simulink model "DAFC_Quadrotor"  (R2025a)
settings: Solver=VariableStepAuto  StartTime=0.0  StopTime=60  RelTol=1e-3
model workspace (MAT data in the model file):
  gamma_a = Simulink.Parameter
  gamma_a.Value = 100
  gamma_a.Complexity = 'real'
  gamma_a.Dimensions = [1 1]
  gamma_a.DataType = 'auto'
  gamma_p = Simulink.Parameter
  gamma_p.Value = 2.5
  gamma_p.Complexity = 'real'
  gamma_p.Dimensions = [1 1]
  gamma_p.DataType = 'auto'
  pna = Simulink.Parameter
  pna.Value = [3; 3.8]
  pna.Complexity = 'real'
  pna.Dimensions = [2 1]
  pna.DataType = 'auto'
  pnp = Simulink.Parameter
  pnp.Value = [5; 5]
  pnp.Complexity = 'real'
  pnp.Dimensions = [2 1]
  pnp.DataType = 'auto'
values from neighbouring files (symbols this model uses):
  gamma_a = 100    [DAFC_Quadrotor.m]
  gamma_p = 2.5    [DAFC_Quadrotor.m]
  pna = [3;3.8]    [DAFC_Quadrotor.m]
  pnp = [5;5]    [DAFC_Quadrotor.m]
libraries: uavutilslib x1
settings Model: SimulationMode=accelerator  Creator=vinh1  LastModifiedBy=vinh1
settings HardwareCC: ProdBitPerPointer=32.0  ProdBitPerSizeT=32.0  ProdBitPerPtrDiffT=32.0  ProdWordSize=32.0  ProdHWDeviceType=Intel->x86-32 (Windows32)

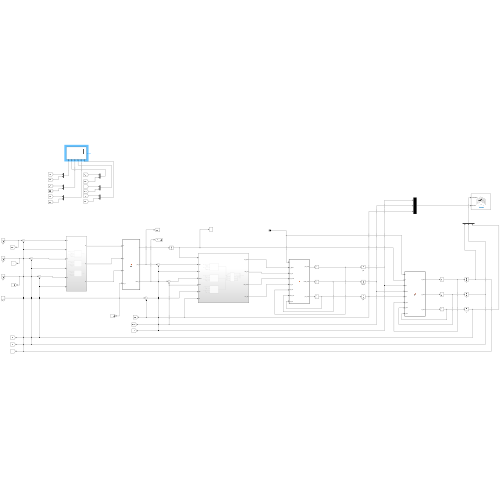
[thumbnail: Simulink's stored preview of the top-level diagram]
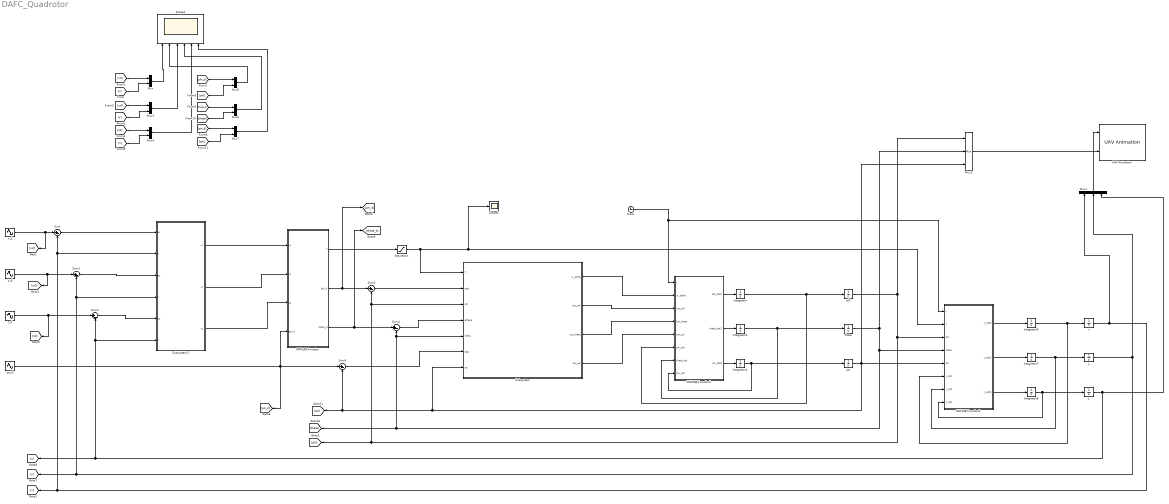
== system DAFC_Quadrotor ==
  Clock : Clock
  Integrator{,2,4,6..8} (6 alike) : Integrator
  MATLAB Function : MATLAB Function  TreatAsAtomicUnit=on
  MATLAB Function1 : MATLAB Function  TreatAsAtomicUnit=on
  MATLAB Function3 : MATLAB Function  TreatAsAtomicUnit=on
  Mux{,3..7} (6 alike) : Mux  Inputs=2
  Mux1 : Mux  Inputs=3
  Mux2 : Mux  Inputs=3
  Saturation : Saturate  UpperLimit=50
  Scope1 : Scope  NumInputPorts=6
      settings: ActiveDisplayString=6  ActiveDisplayYMinimum=-7.5121189989002386E-7  ActiveDisplayYMaximum=4.1251243389959757E-6
  Scope6 : Scope
      settings: ActiveDisplayYMinimum=9.3903851355115471  ActiveDisplayYMaximum=11.595791299111241  DataLoggingVariableName=ScopeData6
  Subsystem : Subsystem
  Subsystem2 : Subsystem
  Sum{,1..5} (6 alike) : Sum  Inputs=|+-
  UAV Animation : uavutilslib/UAV Animation  NumUAV=1  DynamicUAVConfig=off  UAVType=Multirotor  UAVSize=1  UAVColor=[1 0 0]  UAVTrajectoryAlpha=1  InertialZDirection=Up  RotationFormat=Euler ZYX  DrawMarkers=off  SampleTime=-1
  phi : Integrator
  psi : Integrator
  psi_d : Sin  Amplitude=0  Frequency=pi/10  Phase=pi/2  SampleTime=0
  theta : Integrator
  x : Integrator
  x_d : Sin  Amplitude=0.5  Frequency=pi/20  Phase=pi/2  SampleTime=0
  y : Integrator
  y_d : Sin  Amplitude=0.5  Frequency=pi/20  SampleTime=0
  z : Integrator  InitialCondition=2
  z_d : Sin  Amplitude=0.5  Bias=2  Frequency=pi/20  Phase=3*pi/2  SampleTime=0
  wires:
  [psi] -> Mux7/2
  Sum/1 -> Subsystem2/1(ex)
  [phi] -> Mux5/2
  Mux7/1 -> Scope1/6
  Sum2/1 -> Subsystem2/5(ez)
  x_d/1 -> [xd], Sum/1
  Mux6/1 -> Scope1/4
  [zd] -> Mux4/1
  [theta] -> Mux6/2
  Subsystem2/3(uz) -> MATLAB Function/3(uz)
  [yd] -> Mux3/1
  Subsystem2/1(ux) -> MATLAB Function/1(ux)
  [psi_d] -> Mux7/1
  [theta_d] -> Mux6/1
  psi_d/1 -> Sum5/1, [psi_d], MATLAB Function/4(psi_d)
  Subsystem2/2(uy) -> MATLAB Function/2(uy)
  Mux4/1 -> Scope1/5
  [z] -> Mux4/2
  Mux5/1 -> Scope1/2
  [phi_d] -> Mux5/1
  Sum1/1 -> Subsystem2/3(ey)
  Mux3/1 -> Scope1/3
  Mux1/1 -> UAV Animation/1
  [y] -> Mux3/2
  y_d/1 -> Sum1/1, [yd]
  Mux2/1 -> UAV Animation/2
  Mux/1 -> Scope1/1
  z_d/1 -> [zd], Sum2/1
  MATLAB Function1/3(psi_dot2) -> Integrator4/1
  MATLAB Function1/2(theta_dot2) -> Integrator2/1
  MATLAB Function1/1(phi_dot2) -> Integrator/1
  Integrator/1 -> phi/1, MATLAB Function1/6(phi_dot)
  Integrator2/1 -> MATLAB Function1/7(theta_dot), theta/1
  Integrator4/1 -> psi/1, MATLAB Function1/8(psi_dot)
  MATLAB Function/2(phi_d) -> Sum3/1, [phi_d]
  MATLAB Function/3(theta_d) -> [theta_d], Sum4/1
  Subsystem/1(w_alpha) -> MATLAB Function1/2(w_alpha)
  Subsystem/2(tau_phi) -> MATLAB Function1/3(tau_phi)
  Subsystem/3(tau_theta) -> MATLAB Function1/4(tau_theta)
  Subsystem/4(tau_psi) -> MATLAB Function1/5(tau_psi)
  Sum3/1 -> Subsystem/2(ephi)
  Sum4/1 -> Subsystem/4(etheta)
  phi/1 -> Mux2/1, Sum3/2, Subsystem/3(phi), [phi], MATLAB Function3/3(phi)
  theta/1 -> Mux2/2, Sum4/2, Subsystem/5(theta), [theta], MATLAB Function3/4(theta)
  psi/1 -> Mux2/3, MATLAB Function3/5(psi), Sum5/2, [psi], Subsystem/7(psi)
  Sum5/1 -> Subsystem/6(epsi)
  MATLAB Function3/3(z_dot2) -> Integrator8/1
  MATLAB Function3/2(y_dot2) -> Integrator7/1
  MATLAB Function3/1(x_dot2) -> Integrator6/1
  Integrator8/1 -> z/1, MATLAB Function3/8(z_dot)
  Integrator7/1 -> MATLAB Function3/7(y_dot), y/1
  Integrator6/1 -> MATLAB Function3/6(x_dot), x/1
  z/1 -> Mux1/3, [z], Sum2/2, Subsystem2/6(z)
  y/1 -> Sum1/2, Subsystem2/4(y), [y], Mux1/2
  x/1 -> Mux1/1, [x], Sum/2, Subsystem2/2(x)
  Clock/1 -> MATLAB Function3/1(t), MATLAB Function1/1(t)
  Saturation/1 -> Scope6/1, MATLAB Function3/2(T), Subsystem/1(T)
  MATLAB Function/1(T) -> Saturation/1
  [xd] -> Mux/1
  [x] -> Mux/2

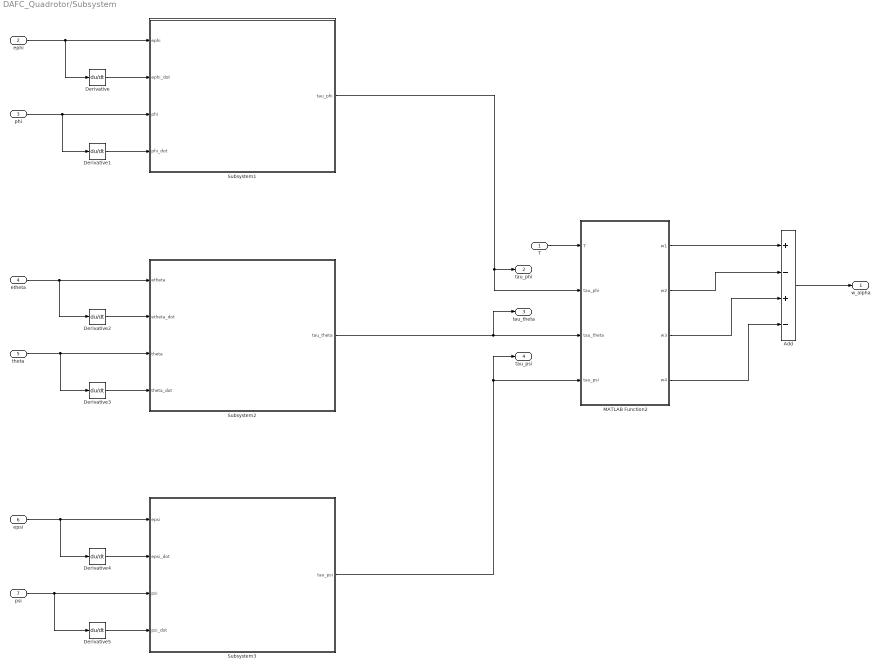
== system DAFC_Quadrotor/Subsystem ==
  T : Inport
  ephi : Inport  Port=2
  phi : Inport  Port=3
  etheta : Inport  Port=4
  theta : Inport  Port=5
  epsi : Inport  Port=6
  psi : Inport  Port=7
  Add : Sum  Inputs=+-+-
  Derivative{,1..5} (6 alike) : Derivative
  MATLAB Function2 : MATLAB Function  TreatAsAtomicUnit=on
  Subsystem1 : Subsystem
  Subsystem2 : Subsystem
  Subsystem3 : Subsystem
  w_alpha : Outport
  tau_phi : Outport  Port=2
  tau_theta : Outport  Port=3
  tau_psi : Outport  Port=4
  wires:
  Derivative4/1 -> Subsystem3/2(epsi_dot)
  Derivative1/1 -> Subsystem1/4(phi_dot)
  Derivative3/1 -> Subsystem2/4(theta_dot)
  Derivative/1 -> Subsystem1/2(ephi_dot)
  Derivative2/1 -> Subsystem2/2(etheta_dot)
  Derivative5/1 -> Subsystem3/4(psi_dot)
  ephi/1 -> Derivative/1, Subsystem1/1(ephi)
  phi/1 -> Subsystem1/3(phi), Derivative1/1
  etheta/1 -> Derivative2/1, Subsystem2/1(etheta)
  theta/1 -> Subsystem2/3(theta), Derivative3/1
  epsi/1 -> Subsystem3/1(epsi), Derivative4/1
  psi/1 -> Derivative5/1, Subsystem3/3(psi)
  MATLAB Function2/3(w3) -> Add/3
  MATLAB Function2/4(w4) -> Add/4
  MATLAB Function2/2(w2) -> Add/2
  MATLAB Function2/1(w1) -> Add/1
  Subsystem1/1(tau_phi) -> tau_phi/1, MATLAB Function2/2(tau_phi)
  Subsystem2/1(tau_theta) -> tau_theta/1, MATLAB Function2/3(tau_theta)
  Subsystem3/1(tau_psi) -> tau_psi/1, MATLAB Function2/4(tau_psi)
  T/1 -> MATLAB Function2/1(T)
  Add/1 -> w_alpha/1

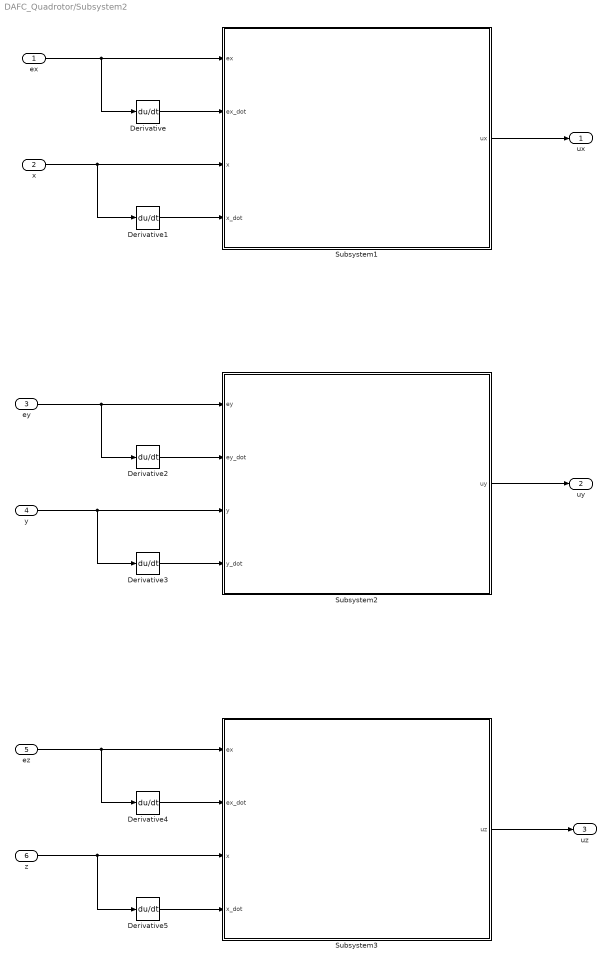
== system DAFC_Quadrotor/Subsystem2 ==
  ex : Inport
  x : Inport  Port=2
  ey : Inport  Port=3
  y : Inport  Port=4
  ez : Inport  Port=5
  z : Inport  Port=6
  Derivative{,1..5} (6 alike) : Derivative
  Subsystem1 : Subsystem
  Subsystem2 : Subsystem
  Subsystem3 : Subsystem
  ux : Outport
  uy : Outport  Port=2
  uz : Outport  Port=3
  wires:
  ex/1 -> Derivative/1, Subsystem1/1(ex)
  Derivative/1 -> Subsystem1/2(ex_dot)
  x/1 -> Subsystem1/3(x), Derivative1/1
  Derivative1/1 -> Subsystem1/4(x_dot)
  ey/1 -> Derivative2/1, Subsystem2/1(ey)
  Derivative2/1 -> Subsystem2/2(ey_dot)
  y/1 -> Subsystem2/3(y), Derivative3/1
  Derivative3/1 -> Subsystem2/4(y_dot)
  ez/1 -> Derivative4/1, Subsystem3/1(ex)
  Derivative4/1 -> Subsystem3/2(ex_dot)
  z/1 -> Derivative5/1, Subsystem3/3(x)
  Derivative5/1 -> Subsystem3/4(x_dot)
  Subsystem1/1(ux) -> ux/1
  Subsystem2/1(uy) -> uy/1
  Subsystem3/1(uz) -> uz/1

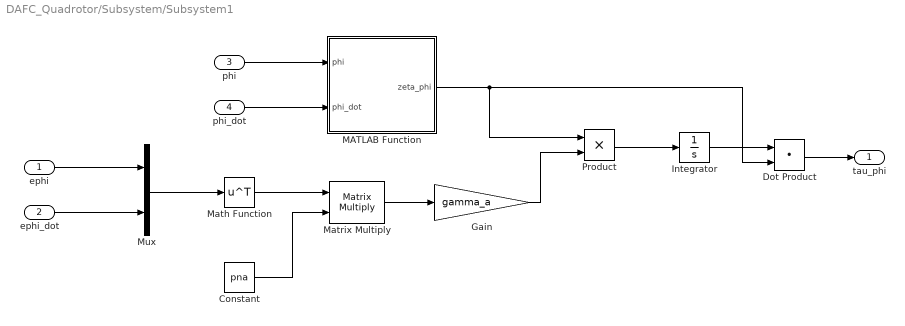
== system DAFC_Quadrotor/Subsystem/Subsystem1 ==
  ephi : Inport
  ephi_dot : Inport  Port=2
  phi : Inport  Port=3
  phi_dot : Inport  Port=4
  Constant : Constant  Value=pna
  Dot Product : DotProduct  OutDataTypeStr=Inherit: Inherit via internal rule
  Gain : Gain  Gain=gamma_a
  Integrator : Integrator
  MATLAB Function : MATLAB Function  TreatAsAtomicUnit=on
  Math Function : Math  Operator=transpose
  Matrix Multiply : Product  Multiplication=Matrix(*)
  Mux : Mux  Inputs=2
  Product : Product
  tau_phi : Outport
  wires:
  Dot Product/1 -> tau_phi/1
  phi_dot/1 -> MATLAB Function/2(phi_dot)
  MATLAB Function/1(zeta_phi) -> Dot Product/2, Product/1
  phi/1 -> MATLAB Function/1(phi)
  Mux/1 -> Math Function/1
  Matrix Multiply/1 -> Gain/1
  Gain/1 -> Product/2
  Constant/1 -> Matrix Multiply/2
  Product/1 -> Integrator/1
  Integrator/1 -> Dot Product/1
  Math Function/1 -> Matrix Multiply/1
  ephi_dot/1 -> Mux/2
  ephi/1 -> Mux/1

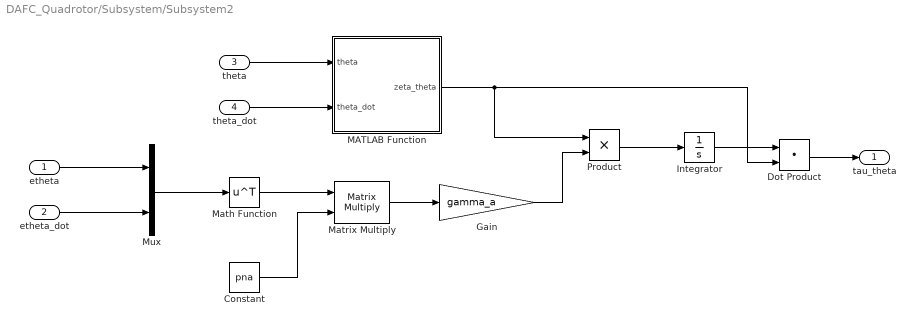
== system DAFC_Quadrotor/Subsystem/Subsystem2 ==
  etheta : Inport
  etheta_dot : Inport  Port=2
  theta : Inport  Port=3
  theta_dot : Inport  Port=4
  Constant : Constant  Value=pna
  Dot Product : DotProduct  OutDataTypeStr=Inherit: Inherit via internal rule
  Gain : Gain  Gain=gamma_a
  Integrator : Integrator
  MATLAB Function : MATLAB Function  TreatAsAtomicUnit=on
  Math Function : Math  Operator=transpose
  Matrix Multiply : Product  Multiplication=Matrix(*)
  Mux : Mux  Inputs=2
  Product : Product
  tau_theta : Outport
  wires:
  etheta/1 -> Mux/1
  etheta_dot/1 -> Mux/2
  Mux/1 -> Math Function/1
  Math Function/1 -> Matrix Multiply/1
  Constant/1 -> Matrix Multiply/2
  Matrix Multiply/1 -> Gain/1
  Gain/1 -> Product/2
  theta/1 -> MATLAB Function/1(theta)
  theta_dot/1 -> MATLAB Function/2(theta_dot)
  Product/1 -> Integrator/1
  MATLAB Function/1(zeta_theta) -> Dot Product/2, Product/1
  Integrator/1 -> Dot Product/1
  Dot Product/1 -> tau_theta/1

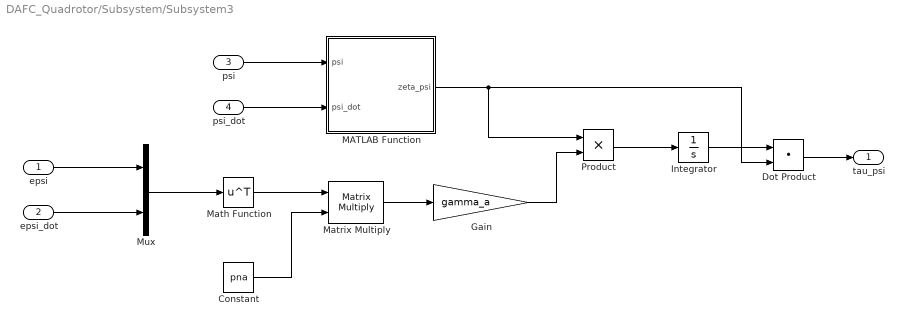
== system DAFC_Quadrotor/Subsystem/Subsystem3 ==
  epsi : Inport
  epsi_dot : Inport  Port=2
  psi : Inport  Port=3
  psi_dot : Inport  Port=4
  Constant : Constant  Value=pna
  Dot Product : DotProduct  OutDataTypeStr=Inherit: Inherit via internal rule
  Gain : Gain  Gain=gamma_a
  Integrator : Integrator
  MATLAB Function : MATLAB Function  TreatAsAtomicUnit=on
  Math Function : Math  Operator=transpose
  Matrix Multiply : Product  Multiplication=Matrix(*)
  Mux : Mux  Inputs=2
  Product : Product
  tau_psi : Outport
  wires:
  Dot Product/1 -> tau_psi/1
  psi_dot/1 -> MATLAB Function/2(psi_dot)
  MATLAB Function/1(zeta_psi) -> Dot Product/2, Product/1
  psi/1 -> MATLAB Function/1(psi)
  Mux/1 -> Math Function/1
  Matrix Multiply/1 -> Gain/1
  Gain/1 -> Product/2
  Constant/1 -> Matrix Multiply/2
  Product/1 -> Integrator/1
  Integrator/1 -> Dot Product/1
  Math Function/1 -> Matrix Multiply/1
  epsi_dot/1 -> Mux/2
  epsi/1 -> Mux/1

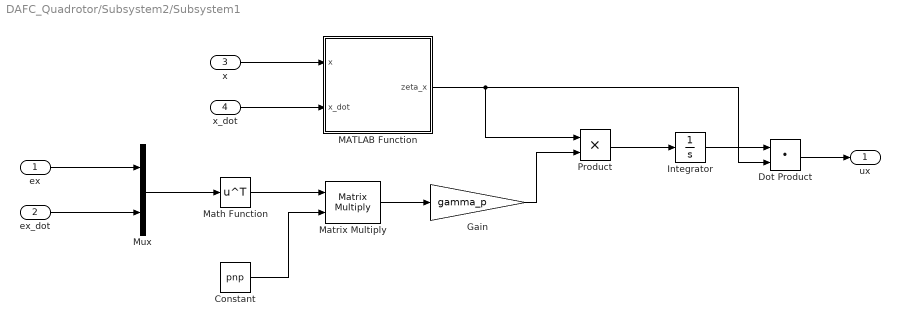
== system DAFC_Quadrotor/Subsystem2/Subsystem1 ==
  ex : Inport
  ex_dot : Inport  Port=2
  x : Inport  Port=3
  x_dot : Inport  Port=4
  Constant : Constant  Value=pnp
  Dot Product : DotProduct  OutDataTypeStr=Inherit: Inherit via internal rule
  Gain : Gain  Gain=gamma_p
  Integrator : Integrator
  MATLAB Function : MATLAB Function  TreatAsAtomicUnit=on
  Math Function : Math  Operator=transpose
  Matrix Multiply : Product  Multiplication=Matrix(*)
  Mux : Mux  Inputs=2
  Product : Product
  ux : Outport
  wires:
  Dot Product/1 -> ux/1
  x_dot/1 -> MATLAB Function/2(x_dot)
  MATLAB Function/1(zeta_x) -> Dot Product/2, Product/1
  x/1 -> MATLAB Function/1(x)
  Mux/1 -> Math Function/1
  Matrix Multiply/1 -> Gain/1
  Gain/1 -> Product/2
  Constant/1 -> Matrix Multiply/2
  Product/1 -> Integrator/1
  Integrator/1 -> Dot Product/1
  Math Function/1 -> Matrix Multiply/1
  ex_dot/1 -> Mux/2
  ex/1 -> Mux/1

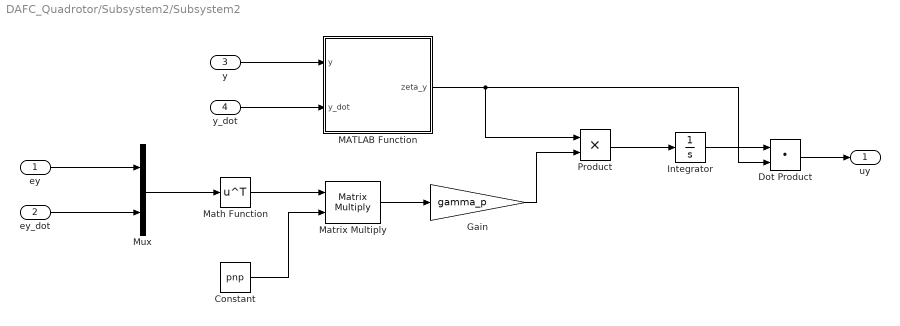
== system DAFC_Quadrotor/Subsystem2/Subsystem2 ==
  ey : Inport
  ey_dot : Inport  Port=2
  y : Inport  Port=3
  y_dot : Inport  Port=4
  Constant : Constant  Value=pnp
  Dot Product : DotProduct  OutDataTypeStr=Inherit: Inherit via internal rule
  Gain : Gain  Gain=gamma_p
  Integrator : Integrator
  MATLAB Function : MATLAB Function  TreatAsAtomicUnit=on
  Math Function : Math  Operator=transpose
  Matrix Multiply : Product  Multiplication=Matrix(*)
  Mux : Mux  Inputs=2
  Product : Product
  uy : Outport
  wires:
  Dot Product/1 -> uy/1
  y_dot/1 -> MATLAB Function/2(y_dot)
  MATLAB Function/1(zeta_y) -> Dot Product/2, Product/1
  y/1 -> MATLAB Function/1(y)
  Mux/1 -> Math Function/1
  Matrix Multiply/1 -> Gain/1
  Gain/1 -> Product/2
  Constant/1 -> Matrix Multiply/2
  Product/1 -> Integrator/1
  Integrator/1 -> Dot Product/1
  Math Function/1 -> Matrix Multiply/1
  ey_dot/1 -> Mux/2
  ey/1 -> Mux/1

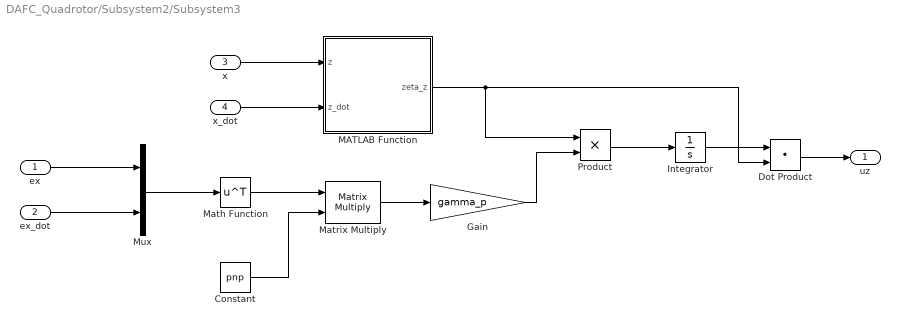
== system DAFC_Quadrotor/Subsystem2/Subsystem3 ==
  ex : Inport
  ex_dot : Inport  Port=2
  x : Inport  Port=3
  x_dot : Inport  Port=4
  Constant : Constant  Value=pnp
  Dot Product : DotProduct  OutDataTypeStr=Inherit: Inherit via internal rule
  Gain : Gain  Gain=gamma_p
  Integrator : Integrator
  MATLAB Function : MATLAB Function  TreatAsAtomicUnit=on
  Math Function : Math  Operator=transpose
  Matrix Multiply : Product  Multiplication=Matrix(*)
  Mux : Mux  Inputs=2
  Product : Product
  uz : Outport
  wires:
  Dot Product/1 -> uz/1
  x_dot/1 -> MATLAB Function/2(z_dot)
  MATLAB Function/1(zeta_z) -> Dot Product/2, Product/1
  x/1 -> MATLAB Function/1(z)
  Mux/1 -> Math Function/1
  Matrix Multiply/1 -> Gain/1
  Gain/1 -> Product/2
  Constant/1 -> Matrix Multiply/2
  Product/1 -> Integrator/1
  Integrator/1 -> Dot Product/1
  Math Function/1 -> Matrix Multiply/1
  ex_dot/1 -> Mux/2
  ex/1 -> Mux/1

== matlab function DAFC_Quadrotor/Subsystem2/Subsystem2/MATLAB Function ==
  data: y input; zeta_y output; y_dot input
function zeta_y = fcn(y, y_dot)

c_y = - 2.5: 1: 2.5;
w_y = 0.5;
c_y_dot = -2: 0.8: 2;
w_y_dot = 0.4;

mu_y = zeros(1, 6);

for i = 1:6
mu_y(i) = exp(-(y - c_y(i))^2 / (2 * w_y^2));
end

mu_y_dot = zeros(1, 6);

for i = 1:6
mu_y_dot(i) = exp(-(y_dot - c_y_dot(i))^2 / (2* w_y_dot^2));
end

zeta_y = zeros(36, 1);
k= 1;

for i = 1:6
    for j = 1:6
    zeta_y(k) = mu_y(i) * mu_y_dot(j);
    k = k + 1;
    end
end

== matlab function DAFC_Quadrotor/Subsystem2/Subsystem3/MATLAB Function ==
  data: z input; zeta_z output; z_dot input
function zeta_z = fcn(z, z_dot)

c_z = 0: 0.6: 3;
w_z = 0.3;
c_z_dot = -1.5: 0.6: 1.5;
w_z_dot = 0.3;

mu_z = zeros(1, 6);

for i = 1:6
mu_z(i) = exp(-(z - c_z(i))^2 / (2 * w_z^2));
end

mu_z_dot = zeros(1, 6);

for i = 1:6
mu_z_dot(i) = exp(-(z_dot - c_z_dot(i))^2 / (2 * w_z_dot^2));
end

zeta_z = zeros(36, 1);
k = 1;

for i = 1:6
    for j = 1:6
    zeta_z(k) = mu_z(i) * mu_z_dot(j);
    k = k + 1;
    end
end

== matlab function DAFC_Quadrotor/Subsystem/MATLAB Function2 ==
  data: T input; w1 output; tau_phi input; tau_theta input; tau_psi input; w2 output; w3 output; w4 output
function [w1, w2, w3, w4] = fcn(T, tau_phi, tau_theta, tau_psi)

k = 2.98e-5 ;
l = 0.25 ;
b = 3.23e-7 ;

w1 = sqrt(max(0,(T/(4*k)) - (tau_theta/(2*k*l)) - (tau_psi/(4*b))));

w2 = sqrt(max(0,(T/(4*k)) - (tau_phi /(2*k*l)) + (tau_psi/(4*b))));

w3 = sqrt(max(0,(T/(4*k)) + (tau_theta/(2*k*l)) - (tau_psi/(4*b))));

w4 = sqrt(max(0,(T/(4*k)) + (tau_phi /(2*k*l)) + (tau_psi/(4*b))));

end

== matlab function DAFC_Quadrotor/MATLAB Function1 ==
  data: t input; w_alpha input; tau_phi input; tau_theta input; tau_psi input; phi_dot2 output; theta_dot2 output; psi_dot2 output; phi_dot input; theta_dot input; psi_dot input
function [phi_dot2, theta_dot2, psi_dot2] = fcn(t, w_alpha, tau_phi, tau_theta, tau_psi, phi_dot, theta_dot, psi_dot)


Ixx = 0.01 ;
Iyy = 0.01 ; 
Izz = 0.0148 ;
Ir = 2.83e-5 ;


dphi = 0.2*sin(2*t) ;
dtheta = 0.2*sin(2*t) ;
dpsi = 0.1*sin(t) ;



phi_dot2 = theta_dot*psi_dot*(Iyy - Izz)/Ixx - theta_dot*w_alpha*Ir/Ixx + tau_phi/Ixx + dphi;

theta_dot2 = phi_dot*psi_dot*(Izz - Ixx)/Iyy + phi_dot*w_alpha*Ir/Iyy + tau_theta/Iyy + dtheta;

psi_dot2 = phi_dot*theta_dot*(Ixx - Iyy)/Izz + tau_psi/Izz + dpsi;

end

== matlab function DAFC_Quadrotor/MATLAB Function ==
  data: ux input; T output; uy input; uz input; psi_d input; phi_d output; theta_d output
function [T, phi_d, theta_d] = fcn(ux, uy, uz, psi_d)

m = 1.121 ;
g = 9.81 ;

T = m*sqrt( (ux)^2 + (uy)^2 + (uz + g)^2);

phi_d = asin((ux*sin(psi_d) - uy*cos(psi_d)) / (T/m));

theta_d = atan((ux*cos(psi_d) + uy*sin(psi_d)) / (uz + g));

== matlab function DAFC_Quadrotor/Subsystem2/Subsystem1/MATLAB Function ==
  data: x input; zeta_x output; x_dot input
function zeta_x = fcn(x, x_dot)

c_x = - 2.5: 1: 2.5;
w_x = 0.5;
c_x_dot = -2: 0.8: 2;
w_x_dot = 0.4;

mu_x = zeros(1, 6);

for i = 1:6
mu_x(i) = exp(-(x - c_x(i))^2 / (2 * w_x^2));
end

mu_x_dot = zeros(1, 6);

for i = 1:6
mu_x_dot(i) = exp(-(x_dot - c_x_dot(i))^2 / (2* w_x_dot^2));
end

zeta_x = zeros(36, 1);
k = 1;

for i = 1:6
    for j = 1:6
    zeta_x(k) = mu_x(i) * mu_x_dot(j);
    k = k + 1;
    end
end

== matlab function DAFC_Quadrotor/MATLAB Function3 ==
  data: t input; T input; phi input; x_dot2 output; theta input; psi input; x_dot input; y_dot2 output; z_dot2 output; y_dot input; z_dot input
function [x_dot2, y_dot2, z_dot2] = fcn(t, T, phi, theta, psi, x_dot, y_dot, z_dot)



Ax = 5.56e-4 ;
Ay = 5.56e-4 ;
Az = 6.35e-4 ;

m = 1.121 ;
g = 9.81 ;


dx = 0.3*sin(t) ;
dy = 0.3*sin(t) ;
dz = 0.1*sin(0.5*t) ;

x_dot2 = (T/m)*( cos(phi)*sin(theta)*cos(psi) + sin(phi)*sin(psi)) - (Ax/m)*x_dot + dx;

y_dot2 = (T/m)*( cos(phi)*sin(theta)*sin(psi) - sin(phi)*cos(psi)) - (Ay/m)*y_dot + dy;

z_dot2 = (T/m)*cos(phi)*cos(theta) - g - (Az/m)*z_dot + dz;

end

== matlab function DAFC_Quadrotor/Subsystem/Subsystem1/MATLAB Function ==
  data: phi input; zeta_phi output; phi_dot input
function zeta_phi = fcn(phi, phi_dot)

c_phi =-pi/9:pi/18:pi/9;
w_phi = pi/36;
c_phi_dot =-1.5:0.6:1.5;
w_phi_dot = 0.3;

mu_phi = zeros(1, 5);

for i = 1:5
mu_phi(i) = exp(-(phi - c_phi(i))^2 / (2 * w_phi^2));
end

mu_phi_dot = zeros(1, 6);

for i = 1:6
mu_phi_dot(i) = exp(-(phi_dot - c_phi_dot(i))^2 / (2 * w_phi_dot^2));
end

zeta_phi = zeros(30, 1);
k= 1;

for i = 1:5
    for j = 1:6
    zeta_phi(k) = mu_phi(i) * mu_phi_dot(j);
    k = k + 1;
    end
end

== matlab function DAFC_Quadrotor/Subsystem/Subsystem2/MATLAB Function ==
  data: theta input; zeta_theta output; theta_dot input
function zeta_theta = fcn(theta, theta_dot)

c_theta =-pi/9:pi/18:pi/9;
w_theta = pi/36;
c_theta_dot =-1.5:0.6:1.5;
w_theta_dot = 0.3;

mu_theta = zeros(1, 5);

for i = 1:5
mu_theta(i) = exp(-(theta - c_theta(i))^2 / (2 * w_theta^2));
end

mu_theta_dot = zeros(1, 6);

for i = 1:6
mu_theta_dot(i) = exp(-(theta_dot - c_theta_dot(i))^2 / (2 * w_theta_dot^2));
end

zeta_theta = zeros(30, 1);
k = 1;

for i = 1:5
    for j = 1:6
    zeta_theta(k) = mu_theta(i) * mu_theta_dot(j);
    k = k + 1;
    end
end

== matlab function DAFC_Quadrotor/Subsystem/Subsystem3/MATLAB Function ==
  data: psi input; zeta_psi output; psi_dot input
function zeta_psi = fcn(psi, psi_dot)

c_psi = -10^-3 : 5*10^-4 : 10^-3;
w_psi = 2.5*10^-4;
c_psi_dot = -0.01 : 4*10^-3 : 0.01;
w_psi_dot = 2*10^-3;

mu_psi = zeros(1, 5);

for i = 1:5
mu_psi(i) = exp(-(psi - c_psi(i))^2 / (2 * w_psi^2));
end

mu_psi_dot = zeros(1, 6);

for i = 1:6
mu_psi_dot(i) =exp(-(psi_dot - c_psi_dot(i))^2 / (2 * w_psi_dot^2));
end

zeta_psi = zeros(30, 1);
k = 1;

for i = 1:5
    for j = 1:6
    zeta_psi(k)= mu_psi(i) * mu_psi_dot(j);
    k = k + 1;
    end
end
